simulink model "boost_converter"  (R2025b)
settings: Solver=ode23t  StartTime=0.1  StopTime=0.5  MaxStep=1e-5  RelTol=1e-3
libraries: nesl_utility x7, fl_lib x5, ee_lib x2, eePwmGenerator x1, simulink x1
settings Model: Creator=Krupal Babariya  LastModifiedBy=Krupal Babariya

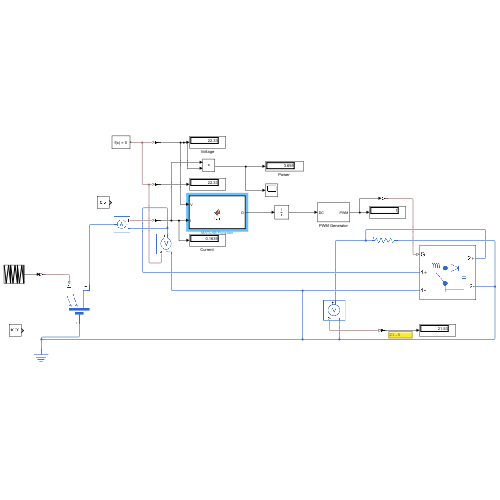
[thumbnail: Simulink's stored preview of the top-level diagram]
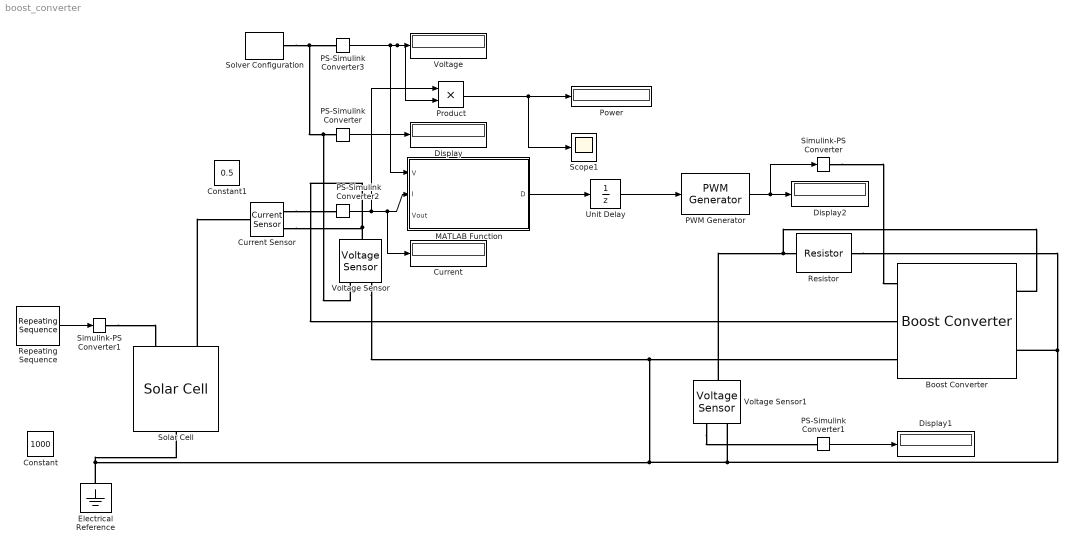
== system boost_converter ==
  Boost Converter : ee_lib/Semiconductors & Converters/Converters/Boost Converter  port_option=ee.enum.controlport.ps  device_type=ee.enum.converters.switchingdevice.mosfet  Vf=0.8 V  Ron=0.001 Ohm  Rds=0.001 Ohm  Goff=1e-5 1/Ohm  Vgt=1 V  Vgt_off=-1 V  Ih=1 A  Vth=6 V  K=0  diode_param=ee.enum.converters.protectiondiode.nodynamics  diode_Vf=0.8 V  diode_Ron=0.001 Ohm  diode_Goff=0.001 1/Ohm  diode_C=50 nF  diode_iRM=-235 A  diode_iF=300 A  diode_idot=-50 A/us  diode_trr_param=ee.enum.converters.diodetrr.trr_factor  diode_trr_factor=3  diode_trr=15 us  diode_Qrr=1500 s*uA  Lf=2 mH  Rl=0 Ohm  Cf=1000e-6 F  Rf=1e-6 Ohm  snubber_type=ee.enum.converters.snubber.exclude  Cs=1e-7 F  Rs=0.1 Ohm  iL_specify=off  iL_priority=High  iL=0 A  iL_nominal_specify=off  iL_nominal_value=1  iL_nominal_unit=A  vc_specify=off  vc_priority=High  vc=0 V  vc_nominal_specify=off  vc_nominal_value=1  vc_nominal_unit=V
      settings: InternalSimscapePortConfiguration="{\"Bottom\":[],\"Left\":[{\"id\":\"G\",\"label\":\"G\",\"type\":\"input\"},{\"id\":\"p1\",\"label\":\"1+\",\"type\":\"foundation.electrical.electrical\"},{\"id\":\"n1\",\"label\":\"1-\",\"type\":\"foundation.electrical.electrical\"}],\"Right\":[{\"id\":\"p2\",\"label\":\"2+\",\"type\":\"foundation.electrical.electrical\"},{\"id\":\"n2\",\"label\":\"2-\",\"type\":\"foundation.electrical.electrical\"}],\"Top\":[]}"
  Constant : Constant  Value=1000
  Constant1 : Constant  Value=0.5
  "Current " : Display
  Current Sensor : fl_lib/Electrical/Electrical Sensors/Current Sensor
  Display : Display
  Display1 : Display
  Display2 : Display
  Electrical Reference : fl_lib/Electrical/Electrical Elements/Electrical Reference
  MATLAB Function : MATLAB Function  TreatAsAtomicUnit=on  SystemSampleTime=0.001
  PS-Simulink Converter{,1..3} (4 alike) : nesl_utility/PS-Simulink Converter  PhysicalDomain=network_engine_domain  SubClassName=ps_output  LeftPortType=input  RightPortType=output  PseudoPeriodic=off  Frequencies=[]  VectorFormat=inherit  Unit=inherit  AffineConversion=off
  PWM Generator : eePwmGenerator/PWM Generator  CarrCount=Up  Tper=1e-4  Tdelay=0  Ts=1e-6
  "Power " : Display
  Product : Product
  Repeating Sequence : simulink/Sources/Repeating Sequence  rep_seq_t=[0 0.5 1.0 1.5]  rep_seq_y=[1000 600 1000 600]
  Resistor : fl_lib/Electrical/Electrical Elements/Resistor  R=150 Ohm  i_specify=off  i_priority=None  i=0 A  i_nominal_specify=off  i_nominal_value=1  i_nominal_unit=A  v_specify=off  v_priority=None  v=0 V  v_nominal_specify=off  v_nominal_value=1  v_nominal_unit=V
  Scope1 : Scope
      settings: ActiveDisplayYMinimum=1.8475347652723314E-7  ActiveDisplayYMaximum=9.8478530382720287E-7
  Simulink-PS Converter : nesl_utility/Simulink-PS Converter  PhysicalDomain=network_engine_domain  SubClassName=ps_input  LeftPortType=input  RightPortType=output  PseudoPeriodic=off  Frequencies=[]  NoiseDistribution=none  NoiseParameters=[]  Unit=V  AffineConversion=off  FilteringAndDerivatives=provide  SimscapeFilterOrder=1  InputFilterTimeConstant=0.001  UdotUserProvided=0
  Simulink-PS Converter1 : nesl_utility/Simulink-PS Converter  PhysicalDomain=network_engine_domain  SubClassName=ps_input  LeftPortType=input  RightPortType=output  PseudoPeriodic=off  Frequencies=[]  NoiseDistribution=none  NoiseParameters=[]  Unit=1  AffineConversion=off  FilteringAndDerivatives=provide  SimscapeFilterOrder=1  InputFilterTimeConstant=0.001  UdotUserProvided=0
  Solar Cell : ee_lib/Sources/Solar Cell  prm=ee.enum.sources.solar_cell_prm.fiveParameter  Isc=8.21 A  Voc=32.9 V  Is=2.66e-5 A  Is2=0 A  Iph=8.21 A  Ir0=1000 W/m^2  ec=1.3  N2=2  Rs=0.221 Ohm  Rp=inf Ohm  N_series=60  N_parallel=1  TIPH1=0 1/K  EG=1.11 eV  TXIS1=3  TXIS2=3  TRS1=0  TRP1=0  Tmeas=25 degC  TFIXED=25 degC  thermal_mass=100 J/K  initial_temperature=25 degC
  Solver Configuration : nesl_utility/Solver Configuration  PhysicalDomain=network_engine_domain  SubClassName=solver  LeftPortType=input  RightPortType=generic  Tones=[]  Harmonics=[]  SimulateNoise=off  Profile=off  UseLocalSampling=off  EnableSwitchedLinearOptims=on  FrequencyDomain=off  UseCCode=off  RelTol=0.001  AbsTol=0.001  MinStep=1e-09  ToWorkspace=off  RevertToSquareIcSolve=off  NumHomotopyIterations=100  PhasorMode=off  PhasorModeNumHarmonics=1  ConsistencySolver=NEWTON_XTOL_AFTER_FTOL  IndexReductionMethod=DerivativeReplacement  DoDC=off  ResidualTolerance=1e-09  ConsistencyTolSource=GLOBAL  ConsistencyAbsTol=0.001  ConsistencyRelTol=0.001  ConsistencyTolFactor=0.001  UseLocalSolver=off  LocalSolverChoice=NE_BACKWARD_EULER_ADVANCER  ResolveIndetEquations=on  FunctionEvalNumThread=1  LocalSolverSampleTime=0.001  DoFixedCost=off  MaxNonlinIter=3  MaxModeIter=2  ComputeImpulses=off  ImpulseIterations=2  LinearAlgebra=auto  LinearAlgebraNumThread=0  EquationFormulation=NE_TIME_EF  DelaysMemoryBudget=1024  AutomaticFiltering=on  FilteringTimeConstant=0.001  PartitionStorageMethod=AS_NEEDED  PartitionMemoryBudget=1024  PartitionMethod=ROBUST  MultibodyUseLocalSolver=off  MultibodyLocalSolverChoice=ODE1  MultibodyLocalSolverSampleTime=0.001
  Unit Delay : UnitDelay  InitialCondition=0.5  SampleTime=-1  HasFrameUpgradeWarning=on
  Voltage : Display
  Voltage Sensor : fl_lib/Electrical/Electrical Sensors/Voltage Sensor
  Voltage Sensor1 : fl_lib/Electrical/Electrical Sensors/Voltage Sensor
  wires:
  PS-Simulink Converter3/1 -> Product/2, Voltage/1, MATLAB Function/1(V)
  PS-Simulink Converter/1 -> Display/1
  PS-Simulink Converter2/1 -> MATLAB Function/2(I), "Current "/1, Product/1
  Product/1 -> "Power "/1, Scope1/1
  MATLAB Function/1(D) -> Unit Delay/1
  Unit Delay/1 -> PWM Generator/1
  PWM Generator/1 -> Display2/1, Simulink-PS Converter/1
  PS-Simulink Converter1/1 -> Display1/1
  Repeating Sequence/1 -> Simulink-PS Converter1/1
  connections:
  Solver Configuration/RConn1 -- Voltage Sensor/RConn1 -- PS-Simulink Converter/LConn1 -- PS-Simulink Converter3/LConn1
  Solar Cell/LConn2 -- Current Sensor/LConn1
  Simulink-PS Converter1/RConn1 -- Solar Cell/LConn1
  Resistor/RConn1 -- Electrical Reference/LConn1 -- Solar Cell/RConn1 -- Boost Converter/LConn3 -- Voltage Sensor/RConn2 -- Voltage Sensor1/RConn2 -- Boost Converter/RConn2
  Current Sensor/RConn1 -- PS-Simulink Converter2/LConn1
  Voltage Sensor1/RConn1 -- PS-Simulink Converter1/LConn1
  Voltage Sensor1/LConn1 -- Boost Converter/RConn1 -- Resistor/LConn1
  Simulink-PS Converter/RConn1 -- Boost Converter/LConn1
  Voltage Sensor/LConn1 -- Current Sensor/RConn2 -- Boost Converter/LConn2

== matlab function boost_converter/MATLAB Function ==
  data: V input; D output; I input; Vout input
function D = mppt_with_protection(V, I, Vout)
% MPPT with Protection - PLAIN TEXT VERSION
% No special characters, only basic ASCII

persistent D_old P_old V_old

% Initialize persistent variables
if isempty(D_old)
    D_old = 0.4;
    P_old = 0;
    V_old = 0;
end

% Protection limits
V_PV_MAX = 33.5;
I_PV_MAX = 9.0;
V_OUT_MAX = 60;

% Display current values (simple format)
fprintf('V=%.2f I=%.2f Vout=%.2f\n', V, I, Vout);

% Check for faults
fault = 0;

if V > V_PV_MAX
    fault = 1;
    fprintf('FAULT: Over-Voltage V=%.2f\n', V);
end

if I > I_PV_MAX
    fault = 1;
    fprintf('FAULT: Over-Current I=%.2f\n', I);
end

if Vout > V_OUT_MAX
    fault = 1;
    fprintf('FAULT: Output OV Vout=%.2f\n', Vout);
end

if fault == 1
    D = 0;
    fprintf('SHUTDOWN - Duty=0\n');
    return;
end

% Normal MPPT operation
step = 0.03;
D_min = 0.1;
D_max = 0.85;

P_new = V * I;

if P_new > P_old && abs(P_new - P_old) > 0.1
    if V > V_old
        D = D_old - step;
    else
        D = D_old + step;
    end
else
    if V > V_old
        D = D_old + step;
    else
        D = D_old - step;
    end
end

D = max(D_min, min(D_max, D));
D_old = D;
P_old = P_new;
V_old = V;

end
